simulink model "Plant_VFD_plus_IM"  (R2021a)
settings: Solver=FixedStepDiscrete  StartTime=0.0  StopTime=5  FixedStep=1e-5  RelTol=1e-3
model workspace (MAT data in the model file):
  Sig = Simulink.Signal
  Sig.DataType = 'auto'
  Sig.Dimensions = -1
  Sig.DimensionsMode = 'auto'
  Sig.Complexity = 'auto'
  Sig.SampleTime = -1
  Sig.SamplingMode = 'auto'
  Sig1 = Simulink.Signal
  Sig1.DataType = 'auto'
  Sig1.Dimensions = -1
  Sig1.DimensionsMode = 'auto'
  Sig1.Complexity = 'auto'
  Sig1.SampleTime = -1
  Sig1.SamplingMode = 'auto'
  Sig2 = Simulink.Signal
  Sig2.DataType = 'auto'
  Sig2.Dimensions = -1
  Sig2.DimensionsMode = 'auto'
  Sig2.Complexity = 'auto'
  Sig2.SampleTime = -1
  Sig2.SamplingMode = 'auto'
  amplitue = 1
  carier_frequency = 16000
  frequency = 400
  x = 90
libraries: spsIGBTDiodeLib x6, spsDiodeLib x4, spsSeriesRLCBranchLib x4, spsabctoAlphaBetaZeroLib x3, spsAsynchronousMachineSIUnitsLib x2, spsCurrentMeasurementLib x2, spsGroundLib x2, simulink x2, spsThreePhaseVIMeasurementLib x2, spsVoltageMeasurementLib x2, spsACVoltageSourceLib x1, spsAlphaBetaZerotoabcLib x1
settings Model: OrderedModelArguments=off  Creator=Mehra  LastModifiedBy=Mehra
settings DebuggingCC: UnconnectedInputMsg=none  UnconnectedOutputMsg=none  UnconnectedLineMsg=none

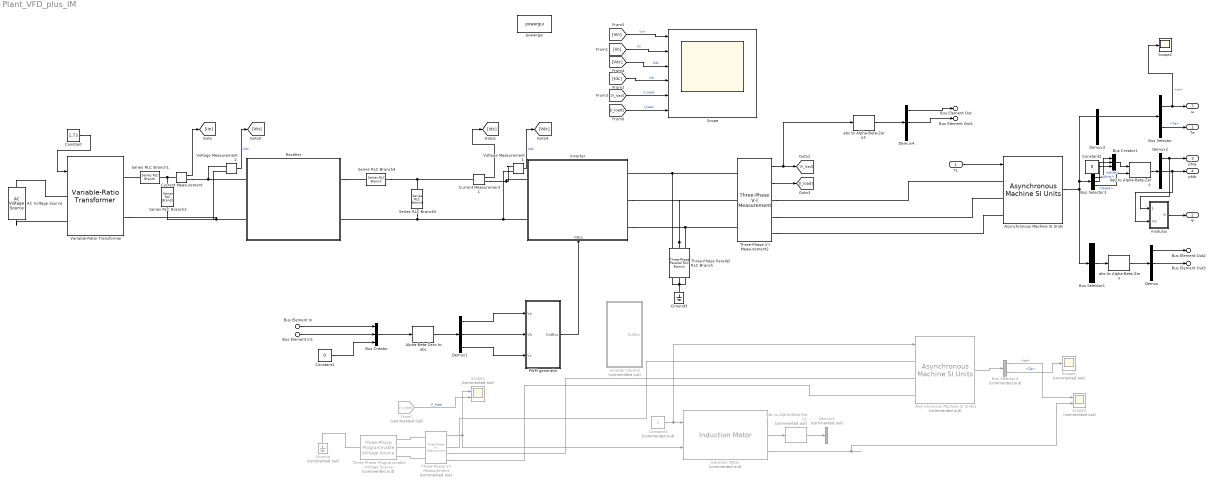
== system Plant_VFD_plus_IM ==
  TL : Inport
  Bus Element In : Inport  Port=2  PortName=Uab  Element=Usa
  Bus Element In1 : Inport  Port=2  PortName=Uab  Element=Usb
  AC Voltage Source : spsACVoltageSourceLib/AC Voltage Source  Amplitude=230  Phase=0  Frequency=50  SampleTime=0  Measurements=None  BusType=swing  Pref=10e3  Qref=0  Qmin=-inf  Qmax=+inf
  Alpha-Beta-Zero to abc : spsAlphaBetaZerotoabcLib/Alpha-Beta-Zero to abc
      settings: SourceProductBaseCode=PS
  Asynchronous Machine SI Units : spsAsynchronousMachineSIUnitsLib/Asynchronous Machine SI Units  RotorType=Squirrel-cage  PresetModel=No  MechanicalLoad=Torque Tm  ShowDetailedParameters=on  ReferenceFrame=Stationary  Units=SI  MeasurementBus=on  NominalParameters=[600 120 17]  VoltageRatio=1  Stator=[5.3 0.365]  Rotor=[3.3 0.375]  Cage1=[0.4155 0.002066]  Cage2=[0.4168 0.0003495]  Lm=0.34  Mechanical=[0.0075 0.005752 2]  PolePairs=2  InitialConditions=[1 0 0 0 0 0.1 0.0366 -0.137]  SimulateSaturation=off  Saturation=[14.03593122, 27.81365428, 53.79336849, 72.68890987, 97.98006896, 148.6815601, 215.7428561, 302.9841135, 428.7778367 ; 230, 322, 414, 460, 506, 552, 598, 644, 690]  LoadFlowParameters=1492000  TsPowergui=0  TsBlock=-1  IterativeModel=Trapezoidal non iterative  IterativeDiscreteModel=Trapezoidal non iterative  Pmec=1.492e+006
  Asynchronous Machine SI Units1 : spsAsynchronousMachineSIUnitsLib/Asynchronous Machine SI Units  Commented=on  RotorType=Squirrel-cage  PresetModel=No  MechanicalLoad=Torque Tm  ShowDetailedParameters=on  ReferenceFrame=Rotor  Units=SI  MeasurementBus=on  NominalParameters=[600 120 17]  VoltageRatio=1  Stator=[5.3 0.365]  Rotor=[3.3 0.375]  Cage1=[0.4155 0.002066]  Cage2=[0.4168 0.0003495]  Lm=0.34  Mechanical=[0.0075 0.005752 2]  PolePairs=2  InitialConditions=[1 0 0 0 0 0.1 0.0366 -0.137]  SimulateSaturation=off  Saturation=[14.03593122, 27.81365428, 53.79336849, 72.68890987, 97.98006896, 148.6815601, 215.7428561, 302.9841135, 428.7778367 ; 230, 322, 414, 460, 506, 552, 598, 644, 690]  LoadFlowParameters=1492000  TsPowergui=0  TsBlock=-1  IterativeModel=Trapezoidal non iterative  IterativeDiscreteModel=Trapezoidal non iterative  Pmec=1.492e+006
  Bus Creator : BusCreator  Inputs=3
  Bus Creator1 : BusCreator  Inputs=3
  Bus Selector : BusSelector  OutputSignals=w,Te
  Bus Selector1 : BusSelector  OutputSignals=ias,ibs,ics  OutputAsBus=on
  Bus Selector3 : BusSelector  OutputSignals=phidr,phiqr,theta
  Bus Selector4 : BusSelector  Commented=on  OutputSignals=w,Te
  Constant : Constant  Value=1.73
  Constant1 : Constant  Value=0
  Constant2 : Constant  Value=0
  Constant3 : Constant  Commented=on
  Current Measurement : spsCurrentMeasurementLib/Current Measurement  PhasorSimulation=off  OutputType=Complex  PSBequivalent=0
  Current Measurement1 : spsCurrentMeasurementLib/Current Measurement  PhasorSimulation=off  OutputType=Complex  PSBequivalent=0
  Demux{,1..4} (5 alike) : Demux  Outputs=3
  Demux5 : Demux  Commented=on  Outputs=3
  From7 : From  Commented=on  GotoTag=V_load
  Ground : spsGroundLib/Ground  Commented=on  LConnTagsString=a
  Ground3 : spsGroundLib/Ground  LConnTagsString=a
  Induction Motor : autolibim/Induction Motor  Commented=on  sim_type=Discrete  Ts=0.00001  port_config=Torque  P=2  Zs=[5.3 0.365]  Zr="[3.3  0.375]"  Lm=0.34  mechanical=[0.0075 0 0]  theta_init=0  omega_init=1  RefBlkName='autolibim/Induction Motor'  aMode=1
      settings: SourceProductBaseCode=PW,DR,MT,UV,VE
  Inverter : Subsystem
      settings: PortSchema="{\"entries\":[{\"content\":{\"sides\":[{\"content\":{\"connectorIds\":[\"LConn1\",\"LConn2\"]},\"type\":\"ConnectorPlacement.EquallySpacedRectSide\",\"uuid\":\"1a5164be-7b1a-4faa-b680-540d002d9225\"},{\"content\":{\"connectorIds\":[\"RConn1\",\"RConn2\",\"RConn3\"],\"side\":\"RIGHT\"},\"type\":\"ConnectorPlacement.EquallySpacedRectSide\",\"uuid\":\"a4ee44e2-5ce1-494c-b26e-cec26737d1ea\"},{\"content\":{\"connectorIds\":[],\"side\":\"TOP\"},\"type\":\"ConnectorPlacement.EquallySpacedRectSide\",\"uuid\":\"a87e43b4-52c7-4077-b0a2-c6057c8abdd1\"},{\"content\":{\"connectorIds\":[\"In1\"],\"side\":\"BOTTOM\"},\"type\":\"ConnectorPlacement.EquallySpacedRectSide\",\"uuid\":\"0d2bfa9e-1afc-4fe0-9ced-0f164dd27f63\"}]},\"type\":\"ConnectorPlacement.EquallySpacedConnector\",\"uuid\":\"c15c5a08-0b96-4dac-87bc-bcfd65a470f3\"}],\"packageUris\":[\"http://schema.mathworks.com/mf0/Connector/R2020b\"],\"version\":\"1.0\"}"
  Inverter Control : Subsystem  Commented=on
  PWM generator : Subsystem
  Rectifier : Subsystem
  Scope : Scope  NumInputPorts=6
  Scope1 : Scope  Commented=on  NumInputPorts=2
  Scope2 : Scope
  Scope3 : Scope  Commented=on  NumInputPorts=2
  Scope4 : Scope  Commented=on
  Series RLC Branch1 : spsSeriesRLCBranchLib/Series RLC Branch  LConnTagsString=__new0  RConnTagsString=__new0  BranchType=L  Resistance=0.1  Inductance=0.01e-6  SetiL0=off  InitialCurrent=0  Capacitance=120e-6  Setx0=off  InitialVoltage=0  Measurements=None
  Series RLC Branch2 : spsSeriesRLCBranchLib/Series RLC Branch  LConnTagsString=__new0  RConnTagsString=__new0  BranchType=C  Resistance=0.1  Inductance=180e-6  SetiL0=off  InitialCurrent=0  Capacitance=100e-6  Setx0=off  InitialVoltage=0  Measurements=None
  Series RLC Branch4 : spsSeriesRLCBranchLib/Series RLC Branch  LConnTagsString=__new0  RConnTagsString=__new0  BranchType=L  Resistance=0.1  Inductance=0.1e-6  SetiL0=off  InitialCurrent=0  Capacitance=120e-6  Setx0=off  InitialVoltage=0  Measurements=None
  Series RLC Branch5 : spsSeriesRLCBranchLib/Series RLC Branch  LConnTagsString=__new0  RConnTagsString=__new0  BranchType=C  Resistance=0.1  Inductance=180e-6  SetiL0=off  InitialCurrent=0  Capacitance=470e-6  Setx0=off  InitialVoltage=0  Measurements=None
  Three-Phase Parallel RLC Branch : spsThreePhaseParallelRLCBranchLib/Three-Phase Parallel RLC Branch  LConnTagsString=A|B|C  RConnTagsString=A|B|C  BranchType=R  Resistance=1000000000  Inductance=1e-3  Capacitance=47e-6  Measurements=None
      settings: SourceProductBaseCode=PS
  Three-Phase Programmable Voltage Source : spsThreePhaseProgrammableVoltageSourceLib/Three-Phase Programmable Voltage Source  Commented=on  PositiveSequence="[120  0 400]"  VariationEntity=None  VariationType=Table of time-amplitude pairs  VariationTypeAlt=Step  VariationStep=0.5  VariationRate=10  VariationMagnitude=0.3  VariationFrequency=2  VariationTiming=[1 2]  VariationPhaseA=off  Amplitudes=[1 0.8 1.2 1.0]  TimeValues=[0 0.1 0.15 0.2]  HarmonicGeneration=off  HarmonicA=[3 0.2 -25 0]  HarmonicB=[2 0.15 35 2]  Timing="[0.05  3]"  BusType=swing  Pref=0  Qref=0  Qmin=-inf  Qmax=inf
  Three-Phase V-I Measurement : spsThreePhaseVIMeasurementLib/Three-Phase V-I Measurement  Commented=on  VoltageMeasurement=phase-to-ground  SetLabelV=off  LabelV=Vabc  Vpu=off  VpuLL=off  CurrentMeasurement=yes  SetLabelI=off  LabelI=Iabc  Ipu=off  Pbase=100e6  Vbase=500e3  OutputType=Complex  PhasorSimulation=off  PSBequivalent=0
  Three-Phase V-I Measurement2 : spsThreePhaseVIMeasurementLib/Three-Phase V-I Measurement  VoltageMeasurement=phase-to-ground  SetLabelV=off  LabelV=Vabc  Vpu=off  VpuLL=off  CurrentMeasurement=yes  SetLabelI=off  LabelI=Iabc  Ipu=off  Pbase=100e6  Vbase=500e3  OutputType=Complex  PhasorSimulation=off  PSBequivalent=0
  Variable-Ratio Transformer : spsVariableRatioTransformerLib/Variable-Ratio Transformer
      settings: SourceProductBaseCode=PS
  Voltage Measurement1 : spsVoltageMeasurementLib/Voltage Measurement  PhasorSimulation=off  OutputType=Complex  PSBequivalent=0
  Voltage Measurement2 : spsVoltageMeasurementLib/Voltage Measurement  PhasorSimulation=off  OutputType=Complex  PSBequivalent=0
  abc to Alpha-Beta-Zero : spsabctoAlphaBetaZeroLib/abc to Alpha-Beta-Zero
      settings: SourceProductBaseCode=PS
  abc to Alpha-Beta-Zero1 : spsabctoAlphaBetaZeroLib/abc to Alpha-Beta-Zero  Commented=on
      settings: SourceProductBaseCode=PS
  abc to Alpha-Beta-Zero3 : spsabctoAlphaBetaZeroLib/abc to Alpha-Beta-Zero
      settings: SourceProductBaseCode=PS
  dq0 to Alpha-Beta-Zero : spsdq0toAlphaBetaZeroLib/dq0 to Alpha-Beta-Zero  Alignment=90 degrees behind phase A axis
      settings: SourceProductBaseCode=PS
  modulus : Subsystem
  powergui : spspowerguiLib/powergui  Priority=1  SimulationMode=Discrete  SampleTime=1e-5  frequency=60  Iterations=50  frequencyindice=50  Pbase=100e6  ErrMax=1e-4  UnitsV=kV  UnitsW=MW  buscounter=0  FunctionMessages=off  echomessages=off  EnableUseOfTLC=off  CurrentSourceSwitches=off  DisableSnubberDevices=off  DisableRonSwitches=off  DisableVfSwitches=off  DisplayEquations=off  AutomaticDiscreteSolvers=off  SolverType=Tustin/Backward Euler (TBE)  Interpol=off  ExternalGateDelay=off  methode=off  Ts=100  x0status=blocks  SPID=on  SwTol=0  HookPort=off  NonlinearTolerance=1e-4  nMaxIteration=100  ContinueOnMaxIteration=off  RestoreLinks=warning  ResistiveCurrentMeasurement=off  Frange=[0:2:500]  Ylog=off  Xlog=on  ShowGrid=off  save=off  variable=ZData  structure=0  ZoomFFT=off  StartTime=0.0  cycles=1  DisplayStyle=1  fundamental=60  FreqAxis=off  MaxFrequency=1000  frequencyindicesteady=1  RmsSteady=1  display=off
  Te : Outport
  Ψ : Outport  Port=2
  phia : Outport  Port=3
  phib : Outport  Port=4
  Bus Element Out : Outport  Port=5  PortName=Us  Element=Usa
  Bus Element Out1 : Outport  Port=5  PortName=Us  Element=Usb
  Bus Element Out2 : Outport  Port=6  PortName=Is  Element=Isa
  Bus Element Out3 : Outport  Port=6  PortName=Is  Element=Isb
  ω : Outport  Port=7
  wires:
  [Iin] -> Scope/2  "Iin"
  [Idc] -> Scope/4  "Idc"
  [Vin] -> Scope/1  "Vin"
  Current Measurement/1 -> [Iin]
  Current Measurement1/1 -> [Idc]
  [Vdc] -> Scope/3  "Vdc"
  Voltage Measurement1/1 -> [Vdc]  "Vdc"
  Voltage Measurement2/1 -> [Vin]  "Vdc"
  Constant/1 -> Variable-Ratio Transformer/1
  [V_load] -> Scope/5  "V_load"
  [I_load] -> Scope/6  "I_load"
  TL/1 -> Asynchronous Machine SI Units/1
  Asynchronous Machine SI Units/1 -> Bus Selector1/1, Bus Selector/1, Bus Selector3/1
  Bus Selector/1 -> ω/1, Scope2/1  "<w>"
  Bus Selector/2 -> Te/1  "<Te>"
  Bus Selector1/1 -> abc to Alpha-Beta-Zero/1
  abc to Alpha-Beta-Zero/1 -> Demux/1
  Bus Creator/1 -> Alpha-Beta-Zero to abc/1
  Bus Element In/1 -> Bus Creator/1
  Bus Element In1/1 -> Bus Creator/2
  Demux1/1 -> PWM generator/1(Va)
  Demux1/2 -> PWM generator/2(Vb)
  Demux1/3 -> PWM generator/3(Vc)
  Bus Creator1/1 -> dq0 to Alpha-Beta-Zero/1
  Demux2/2 -> modulus/2(In2), phib/1
  dq0 to Alpha-Beta-Zero/1 -> Demux2/1
  Demux2/1 -> modulus/1(1), phia/1
  Constant1/1 -> Bus Creator/3
  Three-Phase V-I Measurement/1 -> Scope1/1, Induction Motor/2
  From7/1 -> Scope1/2  "V_load"
  modulus/1(Ψ) -> Ψ/1
  Three-Phase V-I Measurement2/2 -> [I_load]
  Three-Phase V-I Measurement2/1 -> abc to Alpha-Beta-Zero3/1, [V_load]
  PWM generator/1(OutBus) -> Inverter/1(InBus)
  abc to Alpha-Beta-Zero3/1 -> Demux4/1
  Demux4/1 -> Bus Element Out/1
  Demux4/2 -> Bus Element Out1/1
  Alpha-Beta-Zero to abc/1 -> Demux1/1
  Bus Selector3/1 -> Bus Creator1/1  "<phidr>"
  Bus Selector3/2 -> Bus Creator1/2  "<phiqr>"
  Constant2/1 -> Bus Creator1/3
  Bus Selector3/3 -> dq0 to Alpha-Beta-Zero/2  "<theta>"
  Constant3/1 -> Asynchronous Machine SI Units1/1, Induction Motor/1
  Induction Motor/2 -> abc to Alpha-Beta-Zero1/1
  abc to Alpha-Beta-Zero1/1 -> Demux5/1
  Induction Motor/3 -> Scope3/2
  Asynchronous Machine SI Units1/1 -> Bus Selector4/1
  Bus Selector4/1 -> Scope3/1  "<w>"
  Bus Selector4/2 -> Scope4/1  "<Te>"
  Demux/1 -> Bus Element Out2/1
  Demux/2 -> Bus Element Out3/1
  connections:
  Current Measurement/RConn1 -- Voltage Measurement2/LConn1 -- Rectifier/LConn1
  Current Measurement1/RConn1 -- Voltage Measurement1/LConn1 -- Inverter/LConn1
  Rectifier/RConn1 -- Series RLC Branch4/RConn1
  Voltage Measurement2/LConn2 -- Series RLC Branch2/RConn1 -- Variable-Ratio Transformer/RConn2 -- Rectifier/LConn2
  Voltage Measurement1/LConn2 -- Inverter/LConn2 -- Series RLC Branch5/RConn1 -- Rectifier/RConn2
  Three-Phase Parallel RLC Branch/LConn2 -- Inverter/RConn2 -- Three-Phase V-I Measurement2/LConn2
  Current Measurement/LConn1 -- Series RLC Branch2/LConn1 -- Series RLC Branch1/LConn1
  Series RLC Branch4/LConn1 -- Current Measurement1/LConn1 -- Series RLC Branch5/LConn1
  Three-Phase V-I Measurement2/LConn3 -- Inverter/RConn3 -- Three-Phase Parallel RLC Branch/LConn3
  AC Voltage Source/RConn1 -- Variable-Ratio Transformer/LConn1
  AC Voltage Source/LConn1 -- Variable-Ratio Transformer/LConn2
  Ground/LConn1 -- Three-Phase Programmable Voltage Source/LConn1
  Three-Phase V-I Measurement/LConn1 -- Three-Phase Programmable Voltage Source/RConn1
  Three-Phase V-I Measurement/LConn2 -- Three-Phase Programmable Voltage Source/RConn2
  Three-Phase V-I Measurement/LConn3 -- Three-Phase Programmable Voltage Source/RConn3
  Ground3/LConn1 -- Three-Phase Parallel RLC Branch/RConn3 -- Three-Phase Parallel RLC Branch/RConn1 -- Three-Phase Parallel RLC Branch/RConn2
  Three-Phase V-I Measurement2/RConn1 -- Asynchronous Machine SI Units/LConn1
  Three-Phase V-I Measurement2/RConn2 -- Asynchronous Machine SI Units/LConn2
  Three-Phase V-I Measurement2/RConn3 -- Asynchronous Machine SI Units/LConn3
  Three-Phase Parallel RLC Branch/LConn1 -- Three-Phase V-I Measurement2/LConn1 -- Inverter/RConn1
  Series RLC Branch1/RConn1 -- Variable-Ratio Transformer/RConn1
  Three-Phase V-I Measurement/RConn1 -- Asynchronous Machine SI Units1/LConn1
  Three-Phase V-I Measurement/RConn2 -- Asynchronous Machine SI Units1/LConn2
  Three-Phase V-I Measurement/RConn3 -- Asynchronous Machine SI Units1/LConn3

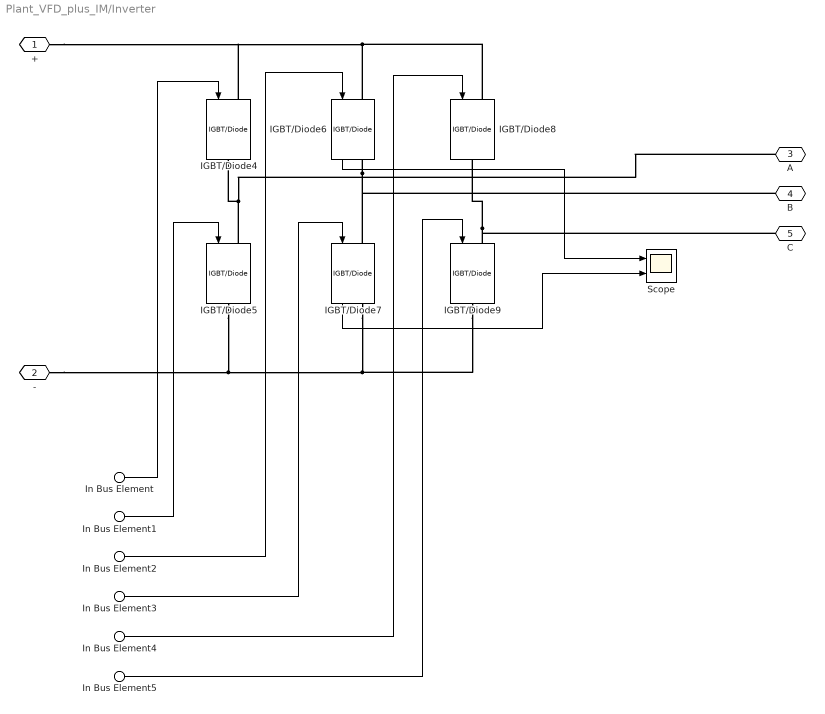
== system Plant_VFD_plus_IM/Inverter ==
  In Bus Element : Inport  PortName=InBus  Element=g1
  In Bus Element1 : Inport  PortName=InBus  Element=g2
  In Bus Element2 : Inport  PortName=InBus  Element=g3
  In Bus Element3 : Inport  PortName=InBus  Element=g4
  In Bus Element4 : Inport  PortName=InBus  Element=g5
  In Bus Element5 : Inport  PortName=InBus  Element=g6
  IGBT/Diode{4..5,8..9} (4 alike) : spsIGBTDiodeLib/IGBT//Diode  Ron=1e-3  Rs=1e5  Cs=inf  Measurements=off
  IGBT/Diode6 : spsIGBTDiodeLib/IGBT//Diode  Ron=1e-3  Rs=1e5  Cs=inf  Measurements=on
  IGBT/Diode7 : spsIGBTDiodeLib/IGBT//Diode  Ron=1e-3  Rs=1e5  Cs=inf  Measurements=on
  Scope : Scope  NumInputPorts=2
  + : PMIOPort  Side=Left
  - : PMIOPort  Port=2  Side=Left
  A : PMIOPort  Port=3  Side=Right
  B : PMIOPort  Port=4  Side=Right
  C : PMIOPort  Port=5  Side=Right
  wires:
  In Bus Element/1 -> IGBT/Diode4/1
  In Bus Element4/1 -> IGBT/Diode8/1
  In Bus Element2/1 -> IGBT/Diode6/1
  IGBT/Diode6/1 -> Scope/1
  IGBT/Diode7/1 -> Scope/2
  In Bus Element1/1 -> IGBT/Diode5/1
  In Bus Element3/1 -> IGBT/Diode7/1
  In Bus Element5/1 -> IGBT/Diode9/1
  connections:
  IGBT/Diode5/LConn1 -- A/RConn1 -- IGBT/Diode4/RConn1
  IGBT/Diode8/LConn1 -- +/RConn1 -- IGBT/Diode4/LConn1 -- IGBT/Diode6/LConn1
  IGBT/Diode6/RConn1 -- IGBT/Diode7/LConn1 -- B/RConn1
  IGBT/Diode5/RConn1 -- -/RConn1 -- IGBT/Diode9/RConn1 -- IGBT/Diode7/RConn1
  IGBT/Diode9/LConn1 -- IGBT/Diode8/RConn1 -- C/RConn1

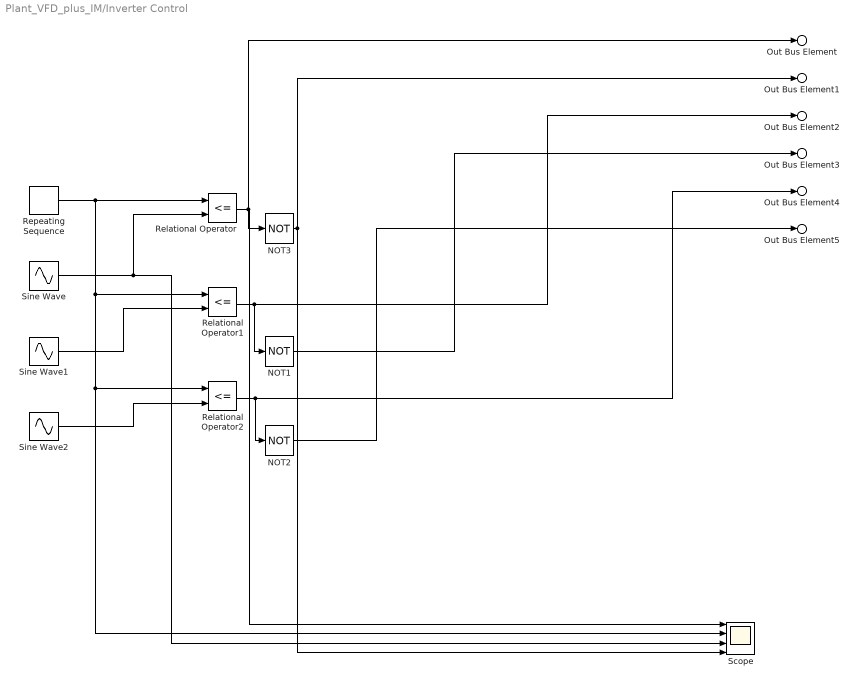
== system Plant_VFD_plus_IM/Inverter Control ==
  NOT1 : Logic  Operator=NOT  IconShape=distinctive  AllPortsSameDT=off  OutDataTypeStr=boolean
  NOT2 : Logic  Operator=NOT  IconShape=distinctive  AllPortsSameDT=off  OutDataTypeStr=boolean
  NOT3 : Logic  Operator=NOT  IconShape=distinctive  AllPortsSameDT=off  OutDataTypeStr=boolean
  Relational Operator : RelationalOperator  Operator=<=  OutDataTypeStr=boolean  RndMeth=Simplest
  Relational Operator1 : RelationalOperator  Operator=<=  OutDataTypeStr=boolean  RndMeth=Simplest
  Relational Operator2 : RelationalOperator  Operator=<=  OutDataTypeStr=boolean  RndMeth=Simplest
  Repeating Sequence : simulink/Sources/Repeating Sequence  rep_seq_t=[0 1/(carier_frequency)]  rep_seq_y=[0 1]
  Scope : Scope  NumInputPorts=4
  Sine Wave : Sin  Amplitude=amplitue  Frequency=2*pi*frequency  SampleTime=0
  Sine Wave1 : Sin  Amplitude=amplitue  Frequency=2*pi*frequency  Phase=2*pi/3  SampleTime=0
  Sine Wave2 : Sin  Amplitude=amplitue  Frequency=2*pi*frequency  Phase=4*pi/3  SampleTime=0
  Out Bus Element : Outport  PortName=OutBus  Element=g1
  Out Bus Element1 : Outport  PortName=OutBus  Element=g2
  Out Bus Element2 : Outport  PortName=OutBus  Element=g3
  Out Bus Element3 : Outport  PortName=OutBus  Element=g4
  Out Bus Element4 : Outport  PortName=OutBus  Element=g5
  Out Bus Element5 : Outport  PortName=OutBus  Element=g6
  wires:
  Sine Wave1/1 -> Relational Operator1/2
  Sine Wave/1 -> Relational Operator/2, Scope/3
  Sine Wave2/1 -> Relational Operator2/2
  Repeating Sequence/1 -> Relational Operator1/1, Scope/2, Relational Operator2/1, Relational Operator/1
  Relational Operator/1 -> NOT3/1, Out Bus Element/1, Scope/1
  NOT3/1 -> Out Bus Element1/1, Scope/4
  Relational Operator1/1 -> NOT1/1, Out Bus Element2/1
  NOT1/1 -> Out Bus Element3/1
  Relational Operator2/1 -> NOT2/1, Out Bus Element4/1
  NOT2/1 -> Out Bus Element5/1

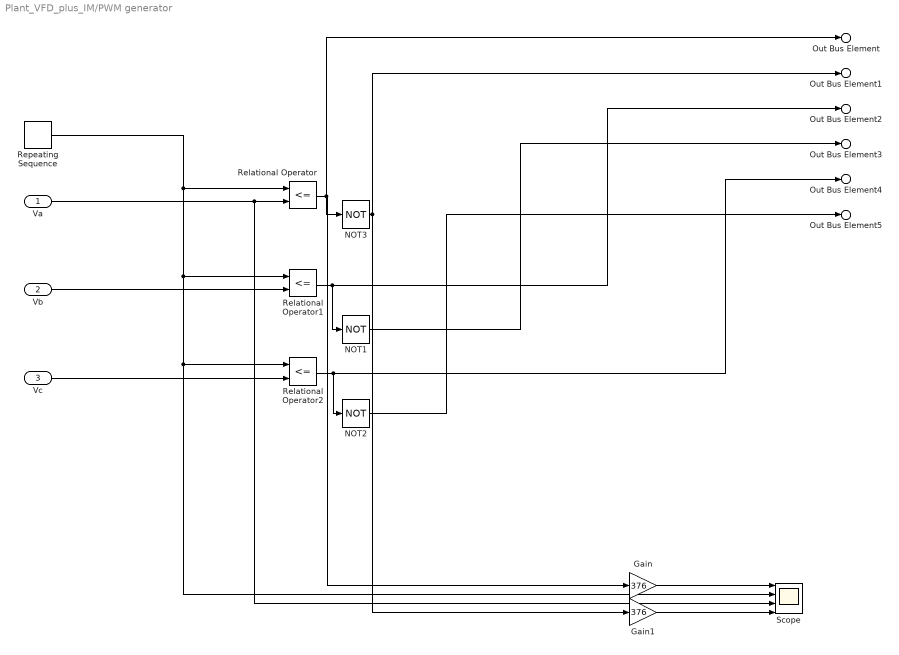
== system Plant_VFD_plus_IM/PWM generator ==
  Va : Inport
  Vb : Inport  Port=2
  Vc : Inport  Port=3
  Gain : Gain  Gain=376
  Gain1 : Gain  Gain=376
  NOT1 : Logic  Operator=NOT  IconShape=distinctive  AllPortsSameDT=off  OutDataTypeStr=boolean
  NOT2 : Logic  Operator=NOT  IconShape=distinctive  AllPortsSameDT=off  OutDataTypeStr=boolean
  NOT3 : Logic  Operator=NOT  IconShape=distinctive  AllPortsSameDT=off  OutDataTypeStr=boolean
  Relational Operator : RelationalOperator  Operator=<=  OutDataTypeStr=boolean  RndMeth=Simplest
  Relational Operator1 : RelationalOperator  Operator=<=  OutDataTypeStr=boolean  RndMeth=Simplest
  Relational Operator2 : RelationalOperator  Operator=<=  OutDataTypeStr=boolean  RndMeth=Simplest
  Repeating Sequence : simulink/Sources/Repeating Sequence  rep_seq_t=[0 1/(carier_frequency)]  rep_seq_y=[0 170]
  Scope : Scope  NumInputPorts=4
  Out Bus Element : Outport  PortName=OutBus  Element=g1
  Out Bus Element1 : Outport  PortName=OutBus  Element=g2
  Out Bus Element2 : Outport  PortName=OutBus  Element=g3
  Out Bus Element3 : Outport  PortName=OutBus  Element=g4
  Out Bus Element4 : Outport  PortName=OutBus  Element=g5
  Out Bus Element5 : Outport  PortName=OutBus  Element=g6
  wires:
  Vb/1 -> Relational Operator1/2
  Va/1 -> Scope/3, Relational Operator/2
  Vc/1 -> Relational Operator2/2
  Repeating Sequence/1 -> Relational Operator1/1, Scope/2, Relational Operator2/1, Relational Operator/1
  Relational Operator/1 -> NOT3/1, Out Bus Element/1, Gain/1
  NOT3/1 -> Out Bus Element1/1, Gain1/1
  Relational Operator1/1 -> NOT1/1, Out Bus Element2/1
  NOT1/1 -> Out Bus Element3/1
  Relational Operator2/1 -> NOT2/1, Out Bus Element4/1
  NOT2/1 -> Out Bus Element5/1
  Gain/1 -> Scope/1
  Gain1/1 -> Scope/4

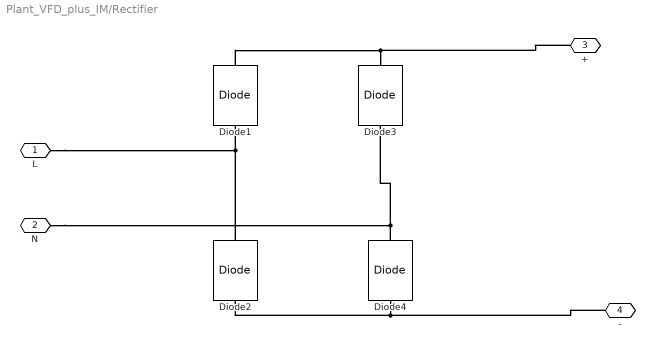
== system Plant_VFD_plus_IM/Rectifier ==
  Diode{1..4} (4 alike) : spsDiodeLib/Diode  Ron=0.001  Lon=0  Vf=0.8  IC=0  UseSnubber=0  Rs=500  Cs=250e-9  Measurements=off
  L : PMIOPort  Side=Left
  N : PMIOPort  Port=2  Side=Left
  + : PMIOPort  Port=3  Side=Right
  - : PMIOPort  Port=4  Side=Right
  connections:
  Diode2/RConn1 -- L/RConn1 -- Diode1/LConn1
  Diode4/RConn1 -- N/RConn1 -- Diode3/LConn1
  Diode1/RConn1 -- +/RConn1 -- Diode3/RConn1
  Diode4/LConn1 -- Diode2/LConn1 -- -/RConn1

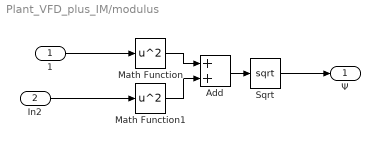
== system Plant_VFD_plus_IM/modulus ==
  1 : Inport
  In2 : Inport  Port=2
  Add : Sum
  Math Function : Math  Operator=square  SaturateOnIntegerOverflow=on
  Math Function1 : Math  Operator=square  SaturateOnIntegerOverflow=on
  Sqrt : Sqrt  SaturateOnIntegerOverflow=on
  Ψ : Outport
  wires:
  Add/1 -> Sqrt/1
  In2/1 -> Math Function1/1
  1/1 -> Math Function/1
  Math Function1/1 -> Add/2
  Math Function/1 -> Add/1
  Sqrt/1 -> Ψ/1
